simulink model "DPTThermalGaNModelSLX"  (R2018a)
settings: Solver=VariableStepAuto  StartTime=0.0  StopTime=8e-6  FixedStep=SampleTime  MinStep=0.5e-12  RelTol=1e-2  AbsTol=1e-9  EnableMultiTasking=on
values from neighbouring files (symbols this model uses):
  LoadCurrent = 15    [DPTThermalGaNModel.m]
  Rd = (3.6/4) * (0.95*0.82*(1 - (-0.0128*(Temp - 25))) * 18.2 / 295) + 1e-4    (= 0.11256119322)    [DPTThermalGaNModel.m]    (also in Thermal_CurrentVoltageGraph.m = (3.6/4) * (0.95*0.82*(1 - (-0.0128*(Temp(TempIndex) - 25))) )
  Rg = 1.5    [DPTThermalGaNModel.m]
  Roff = 2    [DPTThermalGaNModel.m]
  Ron = 10    [DPTThermalGaNModel.m]
  Rs = 3.6 * 0.238 * 0.82 * (1 - (-0.0128*(Temp - 25))) / 295 + 1e-4    (= 0.00629219525424)    [DPTThermalGaNModel.m]    (also in Thermal_CurrentVoltageGraph.m = 3.6 * 0.238 * 0.82 * (1 - (-0.0128*(Temp(TempIndex) - 25))) )
  Rss = 1e-3    (= 0.001)    [DPTThermalGaNModel.m]
  SampleTime = 5e-13    [DPTThermalGaNModel.m]
  Temp = 150    [DPTThermalGaNModel.m]    (also in Thermal_CurrentVoltageGraph.m = 25:25:150)
  Vdc = 400    [DPTThermalGaNModel.m]
  VpulseMax = 6    [DPTThermalGaNModel.m]
  VpulseMin = -3    [DPTThermalGaNModel.m]
undefined symbols (not defined in the file or in its folder): DiscIntNeverNeededParam, DT, T_ON
libraries: elec_lib x62, nesl_utility x33, fl_lib x27, simulink x2
(part 1 of 3)
settings Model: Creator=ugurm  LastModifiedBy=Furkan
settings SolverCC: ShapePreserveControl=EnableAll
settings OptimizationCC: EfficientMapNaN2IntZero=off  LifeSpan=inf
settings DebuggingCC: SFUnexpectedBacktrackingDiag=warning  SFNoUnconditionalDefaultTransitionDiag=warning  SFExecutionAtInitializationDiag=none
settings HardwareCC: TargetBitPerPointer=64  TargetBitPerSizeT=64  TargetBitPerPtrDiffT=64  TargetLongLongMode=on  TargetIntDivRoundTo=Zero  TargetEndianess=LittleEndian  TargetWordSize=64  TargetHWDeviceType=MATLAB Host  ProdEqTarget=off
settings CodeAppCC: MaxIdLength=128  StateflowObjectComments=on
settings GRTTargetCC: TargetLangStandard=C89/C90 (ANSI)  CombineOutputUpdateFcns=off  GRTInterface=on
settings ConfigComp: CovMetricSettings=dw  CovHtmlReporting=on  CovSaveCumulativeToWorkspaceVar=on  CovSaveSingleToWorkspaceVar=on  CovExternalEMLEnable=off
settings SimscapeCC: SimscapeNormalizeSystem=off

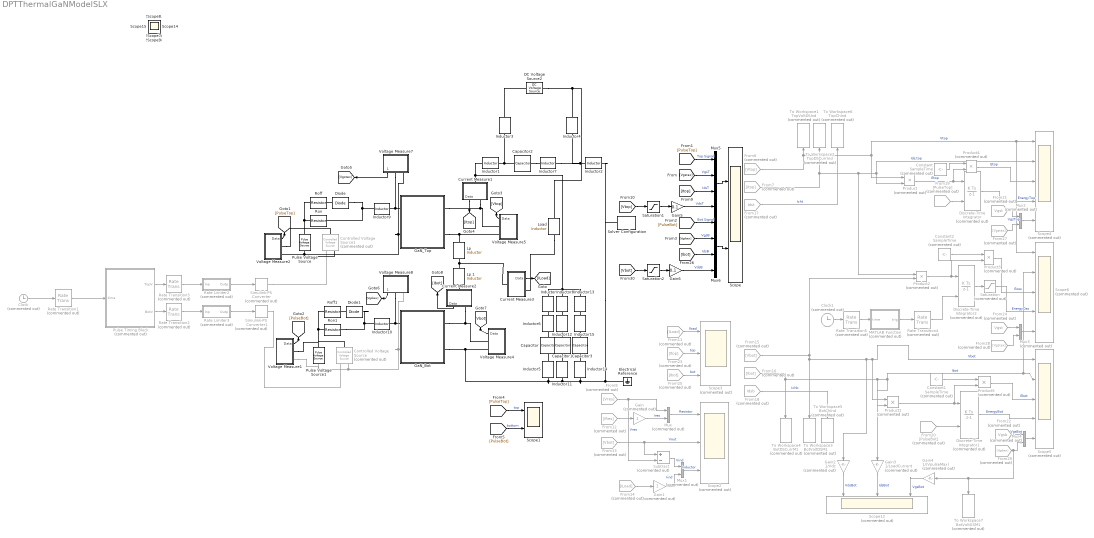
== system DPTThermalGaNModelSLX ==
  Capacitor : elec_lib/Passive Devices/Capacitor  enable_table=0  c=0.1e-6 F  Cvec=[1e-05, 1e-06] F  Vvec=[0, 10] V  CV_table_symmetry=1  C_tol=5  enable_C_tol=0  tol_distribution=1  nSigma=4  r=17.5e-3 Ohm  g=0 1/Ohm  enable_operating_limits=0  operating_limit_action=2  max_working_voltage_range=[-25, 25] V  power_rating=1 W  enable_faults=0  fault_action=1  Cscale_faulted=100  R_faulted=1e-3 Ohm  G_faulted=0 1/Ohm  tau_fault=1e-3 s  enable_temporal_fault=0  t_fault=1 s  enable_behavioral_fault=0  max_permissible_voltage_range=[-100, 100] V  t_fail_on_voltage=1 s  i_specify=off  i_priority=None  i=0 A  i_nominal_specify=off  i_nominal_unit=A  i_nominal_value=1  v_specify=off  v_priority=None  v=0 V  v_nominal_specify=off  v_nominal_unit=V  v_nominal_value=1  vc_specify=on  vc_priority=High  vc=Vdc V  vc_nominal_specify=off  vc_nominal_unit=V  vc_nominal_value=1
  Capacitor1 : elec_lib/Passive Devices/Capacitor  enable_table=0  c=0.1e-6 F  Cvec=[1e-05, 1e-06] F  Vvec=[0, 10] V  CV_table_symmetry=1  C_tol=5  enable_C_tol=0  tol_distribution=1  nSigma=4  r=17.5e-3 Ohm  g=0 1/Ohm  enable_operating_limits=0  operating_limit_action=2  max_working_voltage_range=[-25, 25] V  power_rating=1 W  enable_faults=0  fault_action=1  Cscale_faulted=100  R_faulted=1e-3 Ohm  G_faulted=0 1/Ohm  tau_fault=1e-3 s  enable_temporal_fault=0  t_fault=1 s  enable_behavioral_fault=0  max_permissible_voltage_range=[-100, 100] V  t_fail_on_voltage=1 s  i_specify=off  i_priority=None  i=0 A  i_nominal_specify=off  i_nominal_unit=A  i_nominal_value=1  v_specify=off  v_priority=None  v=0 V  v_nominal_specify=off  v_nominal_unit=V  v_nominal_value=1  vc_specify=on  vc_priority=High  vc=Vdc V  vc_nominal_specify=off  vc_nominal_unit=V  vc_nominal_value=1
  Capacitor2 : elec_lib/Passive Devices/Capacitor  enable_table=0  c=C F  Cvec=[ 1e-5 1e-6 ] F  Vvec=[ 0 10 ] V  CV_table_symmetry=1  C_tol=5  enable_C_tol=0  tol_distribution=1  nSigma=4  r=Resr Ohm  g=0 1/Ohm  enable_operating_limits=0  operating_limit_action=2  max_working_voltage_range=[ -25 25 ] V  power_rating=1 W  enable_faults=0  fault_action=1  Cscale_faulted=100  R_faulted=0.001 Ohm  G_faulted=0 1/Ohm  tau_fault=0.001 s  enable_temporal_fault=0  t_fault=1 s  enable_behavioral_fault=0  max_permissible_voltage_range=[ -100 100 ] V  t_fail_on_voltage=1 s  i_specify=off  i_priority=None  i=0 A  i_nominal_specify=off  i_nominal_unit=A  i_nominal_value=1  v_specify=off  v_priority=None  v=0 V  v_nominal_specify=off  v_nominal_unit=V  v_nominal_value=1  vc_specify=on  vc_priority=High  vc=Vdc V  vc_nominal_specify=off  vc_nominal_unit=V  vc_nominal_value=1
  Capacitor3 : elec_lib/Passive Devices/Capacitor  enable_table=0  c=0.1e-6 F  Cvec=[1e-05, 1e-06] F  Vvec=[0, 10] V  CV_table_symmetry=1  C_tol=5  enable_C_tol=0  tol_distribution=1  nSigma=4  r=17.5e-3 Ohm  g=0 1/Ohm  enable_operating_limits=0  operating_limit_action=2  max_working_voltage_range=[-25, 25] V  power_rating=1 W  enable_faults=0  fault_action=1  Cscale_faulted=100  R_faulted=1e-3 Ohm  G_faulted=0 1/Ohm  tau_fault=1e-3 s  enable_temporal_fault=0  t_fault=1 s  enable_behavioral_fault=0  max_permissible_voltage_range=[-100, 100] V  t_fail_on_voltage=1 s  i_specify=off  i_priority=None  i=0 A  i_nominal_specify=off  i_nominal_unit=A  i_nominal_value=1  v_specify=off  v_priority=None  v=0 V  v_nominal_specify=off  v_nominal_unit=V  v_nominal_value=1  vc_specify=on  vc_priority=High  vc=Vdc V  vc_nominal_specify=off  vc_nominal_unit=V  vc_nominal_value=1
  Clock : Clock  Commented=on
  Clock1 : Clock  Commented=on
  Constant : Constant  Commented=on  Value=SampleTime
  Constant1 : Constant  Commented=on  Value=SampleTime
  Constant2 : Constant  Commented=on  Value=SampleTime
  Controlled Voltage Source : fl_lib/Electrical/Electrical Sources/Controlled Voltage Source  Commented=on
  Controlled Voltage Source1 : fl_lib/Electrical/Electrical Sources/Controlled Voltage Source  Commented=on
  Current Measure1 : Subsystem
  Current Measure2 : Subsystem
  Current Measure3 : Subsystem
  DC Voltage Source2 : elec_lib/Additional Components/SPICE-Compatible Components/Sources/DC Voltage Source  DC=Vdc V
      settings: SourceProductName=Simscape Electronics  SourceProductBaseCode=SN
  Diode : elec_lib/Semiconductor Devices/Diode  ModelType=1  Vf=0.3 V  Ron=15e-3 Ohm  Goff=1e-8 S  Rz=0.3 Ohm  Vz=50 V  C_PWL=5 pF  prmExp=1  I12=[ 0.0137 0.545 ] A  V12=[ 0.6 0.7 ] V  I1=0.0137 A  V1=0.6 V  IS=1e-12 A  ec=1  RS=0.01 Ohm  Tmeas=25 degC  BV=Inf V  C_param=1  CJ0=5 pF  VJ=1 V  Mgrad=0.5  Vvec=[ 0.1 10 100 ] V  Cvec=[ 3.5 1 0.4 ] pF  FC=0.5  Q_param=1  Irrm=-7.15 A  iF=4 A  didt=-750 A/us  trr=115 ns  TT=50 ns  tau=100 ns  T_param=1  IS_T2=1.25e-7 A  I1_T2=0.245 A  V1_T2=0.5 V  Tmeas2=125 degC  EG_param=1  EG=1.11 eV  XTI_param=1  XTI=3  dBVdT=0 V/K  Tdevice=25 degC  i_capacitor_specify=off  i_capacitor_priority=High  i_capacitor=0 A  i_capacitor_nominal_specify=off  i_capacitor_nominal_unit=A  i_capacitor_nominal_value=1  v_capacitor_specify=off  v_capacitor_priority=None  v_capacitor=0 V  v_capacitor_nominal_specify=off  v_capacitor_nominal_unit=V  v_capacitor_nominal_value=1  Rth=[ 0 10 ] K/W  thermal_mass_parameterization=1  thermal_mass=[ 0 1 ] J/K  thermal_time_constant=[ 0 10 ] s  thermal_mass_initial_temperatures=[ 25 25 ] degC
      settings: SourceProductName=Simscape Electronics  SourceProductBaseCode=SN
  Diode1 : elec_lib/Semiconductor Devices/Diode  ModelType=1  Vf=0.3 V  Ron=15e-3 Ohm  Goff=1e-8 S  Rz=0.3 Ohm  Vz=50 V  C_PWL=5 pF  prmExp=1  I12=[ 0.0137 0.545 ] A  V12=[ 0.6 0.7 ] V  I1=0.0137 A  V1=0.6 V  IS=1e-12 A  ec=1  RS=0.01 Ohm  Tmeas=25 degC  BV=Inf V  C_param=1  CJ0=5 pF  VJ=1 V  Mgrad=0.5  Vvec=[ 0.1 10 100 ] V  Cvec=[ 3.5 1 0.4 ] pF  FC=0.5  Q_param=1  Irrm=-7.15 A  iF=4 A  didt=-750 A/us  trr=115 ns  TT=50 ns  tau=100 ns  T_param=1  IS_T2=1.25e-7 A  I1_T2=0.245 A  V1_T2=0.5 V  Tmeas2=125 degC  EG_param=1  EG=1.11 eV  XTI_param=1  XTI=3  dBVdT=0 V/K  Tdevice=25 degC  i_capacitor_specify=off  i_capacitor_priority=High  i_capacitor=0 A  i_capacitor_nominal_specify=off  i_capacitor_nominal_unit=A  i_capacitor_nominal_value=1  v_capacitor_specify=off  v_capacitor_priority=None  v_capacitor=0 V  v_capacitor_nominal_specify=off  v_capacitor_nominal_unit=V  v_capacitor_nominal_value=1  Rth=[ 0 10 ] K/W  thermal_mass_parameterization=1  thermal_mass=[ 0 1 ] J/K  thermal_time_constant=[ 0 10 ] s  thermal_mass_initial_temperatures=[ 25 25 ] degC
      settings: SourceProductName=Simscape Electronics  SourceProductBaseCode=SN
  Discrete-Time Integrator : DiscreteIntegrator  Commented=on  ExternalReset=either  SampleTime=-1  ICPrevOutput=DiscIntNeverNeededParam  ICPrevScaledInput=DiscIntNeverNeededParam
  Discrete-Time Integrator1 : DiscreteIntegrator  Commented=on  ExternalReset=either  SampleTime=-1  ICPrevOutput=DiscIntNeverNeededParam  ICPrevScaledInput=DiscIntNeverNeededParam
  Discrete-Time Integrator2 : DiscreteIntegrator  Commented=on  ExternalReset=either  SampleTime=-1  ICPrevOutput=DiscIntNeverNeededParam  ICPrevScaledInput=DiscIntNeverNeededParam
  Electrical Reference : fl_lib/Electrical/Electrical Elements/Electrical Reference
  From11 : From  Commented=on  GotoTag=ILoad
  From12 : From  Commented=on  GotoTag=IRes
  From13 : From  Commented=on  GotoTag=Vbot
  From14 : From  Commented=on  GotoTag=ILoad
  From15 : From  Commented=on  GotoTag=Vbot
  From16 : From  Commented=on  GotoTag=Ibot
  From17 : From  Commented=on  GotoTag=Idst  TagVisibility=global
  From18 : From  Commented=on  GotoTag=Idsb  TagVisibility=global
  From19 : From  Commented=on  GotoTag=PulseTop
  From20 : From  Commented=on  GotoTag=PulseBot
  From21 : From  Commented=on  GotoTag=Vgst  TagVisibility=global
  From22 : From  Commented=on  GotoTag=Vgsb  TagVisibility=global
  From23 : From  Commented=on  GotoTag=Itop
  From24 : From  Commented=on  GotoTag=Vgst  TagVisibility=global
  From25 : From  Commented=on  GotoTag=Ibot
  From27 : From  Commented=on  GotoTag=Vgstex
  From28 : From  Commented=on  GotoTag=Vgstex
  From29 : From  Commented=on  GotoTag=Vgsbex
  From6 : From  Commented=on  GotoTag=Vtop
  From7 : From  Commented=on  GotoTag=Itop
  From8 : From  Commented=on  GotoTag=Vres
  GaN_Bot : Subsystem
  GaN_Top : Subsystem
  Gain : Gain  Commented=on
  Gain1 : Gain  Commented=on
  Gain2 : Gain  Commented=on  Gain=1/Vdc
  Gain3 : Gain  Commented=on  Gain=1/LoadCurrent
  Gain4 : Gain  Commented=on  Gain=1/(VpulseMax)
  Gain5 : Gain  Gain=0.1
  Gain6 : Gain  Gain=0.1
  Inductor : elec_lib/Passive Devices/Inductor  l=10e-9 H  L_tol=20  enable_L_tol=0  tol_distribution=1  nSigma=4  r=0 Ohm  g=1e-9 1/Ohm  enable_operating_limits=0  operating_limit_action=2  max_working_current=1 A  power_rating=1 W  enable_faults=0  fault_action=1  lambdaPercent=50  k_faulted=0.9999  turnsShort=0  openCct=0  groundShort=0  groundShortG=0 1/Ohm  tau_fault=1e-3 s  enable_temporal_fault=0  t_fault=1 s  enable_behavioral_fault=0  max_permissible_voltage=100 V  n_fail_on_voltage=1  max_permissible_current=1 A  t_fail_on_current=1 s  i_L_specify=off  i_L_priority=High  i_L=0 A  i_L_nominal_specify=off  i_L_nominal_unit=A  i_L_nominal_value=1
      settings: SourceProductName=Simscape Electronics  SourceProductBaseCode=SN
  Inductor1 : elec_lib/Passive Devices/Inductor  l=7.14e-9 H  L_tol=20  enable_L_tol=0  tol_distribution=1  nSigma=4  r=0 Ohm  g=1e-9 1/Ohm  enable_operating_limits=0  operating_limit_action=2  max_working_current=1 A  power_rating=1 W  enable_faults=0  fault_action=1  lambdaPercent=50  k_faulted=0.9999  turnsShort=0  openCct=0  groundShort=0  groundShortG=0 1/Ohm  tau_fault=0.001 s  enable_temporal_fault=0  t_fault=1 s  enable_behavioral_fault=0  max_permissible_voltage=100 V  n_fail_on_voltage=1  max_permissible_current=1 A  t_fail_on_current=1 s  i_L_specify=off  i_L_priority=High  i_L=0 A  i_L_nominal_specify=off  i_L_nominal_unit=A  i_L_nominal_value=1
      settings: SourceProductName=Simscape Electronics  SourceProductBaseCode=SN
  Inductor10 : elec_lib/Passive Devices/Inductor  l=Lgex H  L_tol=20  enable_L_tol=0  tol_distribution=1  nSigma=4  r=0 Ohm  g=1e-9 1/Ohm  enable_operating_limits=0  operating_limit_action=1  max_working_current=1 A  power_rating=1 W  enable_faults=0  fault_action=1  lambdaPercent=50  k_faulted=0.9999  turnsShort=0  openCct=0  groundShort=0  groundShortG=0 1/Ohm  tau_fault=0.001 s  enable_temporal_fault=0  t_fault=1 s  enable_behavioral_fault=0  max_permissible_voltage=100 V  n_fail_on_voltage=1  max_permissible_current=1 A  t_fail_on_current=1 s  i_L_specify=on  i_L_priority=High  i_L=0 A  i_L_nominal_specify=off  i_L_nominal_unit=A  i_L_nominal_value=1
      settings: SourceProductName=Simscape Electronics  SourceProductBaseCode=SN
  Inductor11 : elec_lib/Passive Devices/Inductor  l=12e-9 H  L_tol=20  enable_L_tol=0  tol_distribution=1  nSigma=4  r=0 Ohm  g=1e-9 1/Ohm  enable_operating_limits=0  operating_limit_action=2  max_working_current=1 A  power_rating=1 W  enable_faults=0  fault_action=1  lambdaPercent=50  k_faulted=0.9999  turnsShort=0  openCct=0  groundShort=0  groundShortG=0 1/Ohm  tau_fault=1e-3 s  enable_temporal_fault=0  t_fault=1 s  enable_behavioral_fault=0  max_permissible_voltage=100 V  n_fail_on_voltage=1  max_permissible_current=1 A  t_fail_on_current=1 s  i_L_specify=off  i_L_priority=High  i_L=0 A  i_L_nominal_specify=off  i_L_nominal_unit=A  i_L_nominal_value=1
      settings: SourceProductName=Simscape Electronics  SourceProductBaseCode=SN
  Inductor12 : elec_lib/Passive Devices/Inductor  l=0.75e-9 H  L_tol=20  enable_L_tol=0  tol_distribution=1  nSigma=4  r=0 Ohm  g=1e-9 1/Ohm  enable_operating_limits=0  operating_limit_action=2  max_working_current=1 A  power_rating=1 W  enable_faults=0  fault_action=1  lambdaPercent=50  k_faulted=0.9999  turnsShort=0  openCct=0  groundShort=0  groundShortG=0 1/Ohm  tau_fault=1e-3 s  enable_temporal_fault=0  t_fault=1 s  enable_behavioral_fault=0  max_permissible_voltage=100 V  n_fail_on_voltage=1  max_permissible_current=1 A  t_fail_on_current=1 s  i_L_specify=off  i_L_priority=High  i_L=0 A  i_L_nominal_specify=off  i_L_nominal_unit=A  i_L_nominal_value=1
      settings: SourceProductName=Simscape Electronics  SourceProductBaseCode=SN
  Inductor13 : elec_lib/Passive Devices/Inductor  l=10e-9 H  L_tol=20  enable_L_tol=0  tol_distribution=1  nSigma=4  r=0 Ohm  g=1e-9 1/Ohm  enable_operating_limits=0  operating_limit_action=2  max_working_current=1 A  power_rating=1 W  enable_faults=0  fault_action=1  lambdaPercent=50  k_faulted=0.9999  turnsShort=0  openCct=0  groundShort=0  groundShortG=0 1/Ohm  tau_fault=1e-3 s  enable_temporal_fault=0  t_fault=1 s  enable_behavioral_fault=0  max_permissible_voltage=100 V  n_fail_on_voltage=1  max_permissible_current=1 A  t_fail_on_current=1 s  i_L_specify=off  i_L_priority=High  i_L=0 A  i_L_nominal_specify=off  i_L_nominal_unit=A  i_L_nominal_value=1
      settings: SourceProductName=Simscape Electronics  SourceProductBaseCode=SN
  Inductor14 : elec_lib/Passive Devices/Inductor  l=12e-9 H  L_tol=20  enable_L_tol=0  tol_distribution=1  nSigma=4  r=0 Ohm  g=1e-9 1/Ohm  enable_operating_limits=0  operating_limit_action=2  max_working_current=1 A  power_rating=1 W  enable_faults=0  fault_action=1  lambdaPercent=50  k_faulted=0.9999  turnsShort=0  openCct=0  groundShort=0  groundShortG=0 1/Ohm  tau_fault=1e-3 s  enable_temporal_fault=0  t_fault=1 s  enable_behavioral_fault=0  max_permissible_voltage=100 V  n_fail_on_voltage=1  max_permissible_current=1 A  t_fail_on_current=1 s  i_L_specify=off  i_L_priority=High  i_L=0 A  i_L_nominal_specify=off  i_L_nominal_unit=A  i_L_nominal_value=1
      settings: SourceProductName=Simscape Electronics  SourceProductBaseCode=SN
  Inductor15 : elec_lib/Passive Devices/Inductor  l=0.75e-9 H  L_tol=20  enable_L_tol=0  tol_distribution=1  nSigma=4  r=0 Ohm  g=1e-9 1/Ohm  enable_operating_limits=0  operating_limit_action=2  max_working_current=1 A  power_rating=1 W  enable_faults=0  fault_action=1  lambdaPercent=50  k_faulted=0.9999  turnsShort=0  openCct=0  groundShort=0  groundShortG=0 1/Ohm  tau_fault=1e-3 s  enable_temporal_fault=0  t_fault=1 s  enable_behavioral_fault=0  max_permissible_voltage=100 V  n_fail_on_voltage=1  max_permissible_current=1 A  t_fail_on_current=1 s  i_L_specify=off  i_L_priority=High  i_L=0 A  i_L_nominal_specify=off  i_L_nominal_unit=A  i_L_nominal_value=1
      settings: SourceProductName=Simscape Electronics  SourceProductBaseCode=SN
  Inductor2 : elec_lib/Passive Devices/Inductor  l=5.658e-9 H  L_tol=20  enable_L_tol=0  tol_distribution=1  nSigma=4  r=0.025 Ohm  g=1e-9 1/Ohm  enable_operating_limits=0  operating_limit_action=2  max_working_current=1 A  power_rating=1 W  enable_faults=0  fault_action=1  lambdaPercent=50  k_faulted=0.9999  turnsShort=0  openCct=0  groundShort=0  groundShortG=0 1/Ohm  tau_fault=0.001 s  enable_temporal_fault=0  t_fault=1 s  enable_behavioral_fault=0  max_permissible_voltage=100 V  n_fail_on_voltage=1  max_permissible_current=1 A  t_fail_on_current=1 s  i_L_specify=off  i_L_priority=None  i_L=0 A  i_L_nominal_specify=off  i_L_nominal_unit=A  i_L_nominal_value=1
      settings: SourceProductName=Simscape Electronics  SourceProductBaseCode=SN
  Inductor3 : elec_lib/Passive Devices/Inductor  l=29.8e-9 H  L_tol=20  enable_L_tol=0  tol_distribution=1  nSigma=4  r=0 Ohm  g=1e-9 1/Ohm  enable_operating_limits=0  operating_limit_action=2  max_working_current=1 A  power_rating=1 W  enable_faults=0  fault_action=1  lambdaPercent=50  k_faulted=0.9999  turnsShort=0  openCct=0  groundShort=0  groundShortG=0 1/Ohm  tau_fault=0.001 s  enable_temporal_fault=0  t_fault=1 s  enable_behavioral_fault=0  max_permissible_voltage=100 V  n_fail_on_voltage=1  max_permissible_current=1 A  t_fail_on_current=1 s  i_L_specify=on  i_L_priority=High  i_L=0 A  i_L_nominal_specify=off  i_L_nominal_unit=A  i_L_nominal_value=1
      settings: SourceProductName=Simscape Electronics  SourceProductBaseCode=SN
  Inductor4 : elec_lib/Passive Devices/Inductor  l=48.6e-9 H  L_tol=20  enable_L_tol=0  tol_distribution=1  nSigma=4  r=0 Ohm  g=1e-9 1/Ohm  enable_operating_limits=0  operating_limit_action=2  max_working_current=1 A  power_rating=1 W  enable_faults=0  fault_action=1  lambdaPercent=50  k_faulted=0.9999  turnsShort=0  openCct=0  groundShort=0  groundShortG=0 1/Ohm  tau_fault=0.001 s  enable_temporal_fault=0  t_fault=1 s  enable_behavioral_fault=0  max_permissible_voltage=100 V  n_fail_on_voltage=1  max_permissible_current=1 A  t_fail_on_current=1 s  i_L_specify=on  i_L_priority=High  i_L=0 A  i_L_nominal_specify=off  i_L_nominal_unit=A  i_L_nominal_value=1
      settings: SourceProductName=Simscape Electronics  SourceProductBaseCode=SN
  Inductor5 : elec_lib/Passive Devices/Inductor  l=12e-9 H  L_tol=20  enable_L_tol=0  tol_distribution=1  nSigma=4  r=0 Ohm  g=1e-9 1/Ohm  enable_operating_limits=0  operating_limit_action=2  max_working_current=1 A  power_rating=1 W  enable_faults=0  fault_action=1  lambdaPercent=50  k_faulted=0.9999  turnsShort=0  openCct=0  groundShort=0  groundShortG=0 1/Ohm  tau_fault=1e-3 s  enable_temporal_fault=0  t_fault=1 s  enable_behavioral_fault=0  max_permissible_voltage=100 V  n_fail_on_voltage=1  max_permissible_current=1 A  t_fail_on_current=1 s  i_L_specify=off  i_L_priority=High  i_L=0 A  i_L_nominal_specify=off  i_L_nominal_unit=A  i_L_nominal_value=1
      settings: SourceProductName=Simscape Electronics  SourceProductBaseCode=SN
  Inductor6 : elec_lib/Passive Devices/Inductor  l=0.75e-9 H  L_tol=20  enable_L_tol=0  tol_distribution=1  nSigma=4  r=0 Ohm  g=1e-9 1/Ohm  enable_operating_limits=0  operating_limit_action=2  max_working_current=1 A  power_rating=1 W  enable_faults=0  fault_action=1  lambdaPercent=50  k_faulted=0.9999  turnsShort=0  openCct=0  groundShort=0  groundShortG=0 1/Ohm  tau_fault=1e-3 s  enable_temporal_fault=0  t_fault=1 s  enable_behavioral_fault=0  max_permissible_voltage=100 V  n_fail_on_voltage=1  max_permissible_current=1 A  t_fail_on_current=1 s  i_L_specify=off  i_L_priority=High  i_L=0 A  i_L_nominal_specify=off  i_L_nominal_unit=A  i_L_nominal_value=1
      settings: SourceProductName=Simscape Electronics  SourceProductBaseCode=SN
  Inductor7 : elec_lib/Passive Devices/Inductor  l=19e-9 H  L_tol=20  enable_L_tol=0  tol_distribution=1  nSigma=4  r=0 Ohm  g=1e-9 1/Ohm  enable_operating_limits=0  operating_limit_action=2  max_working_current=1 A  power_rating=1 W  enable_faults=0  fault_action=1  lambdaPercent=50  k_faulted=0.9999  turnsShort=0  openCct=0  groundShort=0  groundShortG=0 1/Ohm  tau_fault=0.001 s  enable_temporal_fault=0  t_fault=1 s  enable_behavioral_fault=0  max_permissible_voltage=100 V  n_fail_on_voltage=1  max_permissible_current=1 A  t_fail_on_current=1 s  i_L_specify=on  i_L_priority=High  i_L=0 A  i_L_nominal_specify=off  i_L_nominal_unit=A  i_L_nominal_value=1
      settings: SourceProductName=Simscape Electronics  SourceProductBaseCode=SN
  Inductor8 : elec_lib/Passive Devices/Inductor  l=10e-9 H  L_tol=20  enable_L_tol=0  tol_distribution=1  nSigma=4  r=0 Ohm  g=1e-9 1/Ohm  enable_operating_limits=0  operating_limit_action=2  max_working_current=1 A  power_rating=1 W  enable_faults=0  fault_action=1  lambdaPercent=50  k_faulted=0.9999  turnsShort=0  openCct=0  groundShort=0  groundShortG=0 1/Ohm  tau_fault=1e-3 s  enable_temporal_fault=0  t_fault=1 s  enable_behavioral_fault=0  max_permissible_voltage=100 V  n_fail_on_voltage=1  max_permissible_current=1 A  t_fail_on_current=1 s  i_L_specify=off  i_L_priority=High  i_L=0 A  i_L_nominal_specify=off  i_L_nominal_unit=A  i_L_nominal_value=1
      settings: SourceProductName=Simscape Electronics  SourceProductBaseCode=SN
  Inductor9 : elec_lib/Passive Devices/Inductor  l=Lgex H  L_tol=20  enable_L_tol=0  tol_distribution=1  nSigma=4  r=0 Ohm  g=1e-9 1/Ohm  enable_operating_limits=0  operating_limit_action=1  max_working_current=1 A  power_rating=1 W  enable_faults=0  fault_action=1  lambdaPercent=50  k_faulted=0.9999  turnsShort=0  openCct=0  groundShort=0  groundShortG=0 1/Ohm  tau_fault=0.001 s  enable_temporal_fault=0  t_fault=1 s  enable_behavioral_fault=0  max_permissible_voltage=100 V  n_fail_on_voltage=1  max_permissible_current=1 A  t_fail_on_current=1 s  i_L_specify=on  i_L_priority=High  i_L=0 A  i_L_nominal_specify=off  i_L_nominal_unit=A  i_L_nominal_value=1
      settings: SourceProductName=Simscape Electronics  SourceProductBaseCode=SN
  Load : elec_lib/Passive Devices/Inductor  l=Lload H  L_tol=20  enable_L_tol=0  tol_distribution=1  nSigma=4  r=0 Ohm  g=1e-9 1/Ohm  enable_operating_limits=0  operating_limit_action=2  max_working_current=1 A  power_rating=1 W  enable_faults=0  fault_action=1  lambdaPercent=50  k_faulted=0.9999  turnsShort=0  openCct=0  groundShort=0  groundShortG=0 1/Ohm  tau_fault=0.001 s  enable_temporal_fault=0  t_fault=1 s  enable_behavioral_fault=0  max_permissible_voltage=100 V  n_fail_on_voltage=1  max_permissible_current=1 A  t_fail_on_current=1 s  i_L_specify=on  i_L_priority=High  i_L=InitialCurrent A  i_L_nominal_specify=off  i_L_nominal_unit=A  i_L_nominal_value=1
      settings: SourceProductName=Simscape Electronics  SourceProductBaseCode=SN
  "Lp " : elec_lib/Passive Devices/Inductor  l=3.724e-9 H  L_tol=20  enable_L_tol=0  tol_distribution=1  nSigma=4  r=0 Ohm  g=1e-9 1/Ohm  enable_operating_limits=0  operating_limit_action=2  max_working_current=1 A  power_rating=1 W  enable_faults=0  fault_action=1  lambdaPercent=50  k_faulted=0.9999  turnsShort=0  openCct=0  groundShort=0  groundShortG=0 1/Ohm  tau_fault=0.001 s  enable_temporal_fault=0  t_fault=1 s  enable_behavioral_fault=0  max_permissible_voltage=100 V  n_fail_on_voltage=1  max_permissible_current=1 A  t_fail_on_current=1 s  i_L_specify=off  i_L_priority=High  i_L=CurrDSTop A  i_L_nominal_specify=off  i_L_nominal_unit=A  i_L_nominal_value=1
      settings: SourceProductName=Simscape Electronics  SourceProductBaseCode=SN
  Lp 1 : elec_lib/Passive Devices/Inductor  l=3.724e-9 H  L_tol=20  enable_L_tol=0  tol_distribution=1  nSigma=4  r=0 Ohm  g=1e-9 1/Ohm  enable_operating_limits=0  operating_limit_action=2  max_working_current=1 A  power_rating=1 W  enable_faults=0  fault_action=1  lambdaPercent=50  k_faulted=0.9999  turnsShort=0  openCct=0  groundShort=0  groundShortG=0 1/Ohm  tau_fault=0.001 s  enable_temporal_fault=0  t_fault=1 s  enable_behavioral_fault=0  max_permissible_voltage=100 V  n_fail_on_voltage=1  max_permissible_current=1 A  t_fail_on_current=1 s  i_L_specify=off  i_L_priority=High  i_L=CurrDSTop A  i_L_nominal_specify=off  i_L_nominal_unit=A  i_L_nominal_value=1
      settings: SourceProductName=Simscape Electronics  SourceProductBaseCode=SN
  MATLAB Function : MATLAB Function  Commented=on  TreatAsAtomicUnit=on  SystemSampleTime=1e-10
  Mux{,1..4} (5 alike) : Mux  Commented=on  Inputs=2
  Mux5 : Mux
  Mux6 : Mux
  Product{,1..5} (6 alike) : Product  Commented=on
  Pulse Timing Block : MATLAB Function  Commented=on  TreatAsAtomicUnit=on  SystemSampleTime=1e-9
  Pulse Voltage Source : elec_lib/Additional Components/SPICE-Compatible Components/Sources/Pulse Voltage Source  V1=VpulseMin V  V2=VpulseMax V  TD=DT s  TR=RiseTime s  TF=FallTime s  PW=T_ON-2*DT s  PER=T_P s
      settings: SourceProductName=Simscape Electronics  SourceProductBaseCode=SN
  Pulse Voltage Source1 : elec_lib/Additional Components/SPICE-Compatible Components/Sources/Pulse Voltage Source  V1=VpulseMax V  V2=VpulseMin V  TD=0 s  TR=RiseTime s  TF=FallTime s  PW=T_ON s  PER=T_P s
      settings: SourceProductName=Simscape Electronics  SourceProductBaseCode=SN
  Rate Limiter2 : Subsystem  Commented=on
  Rate Limiter3 : Subsystem  Commented=on
  Rate Transition1 : RateTransition  Commented=on  OutPortSampleTime=1e-9
  Rate Transition2 : RateTransition  Commented=on  OutPortSampleTime=SampleTime
  Rate Transition3 : RateTransition  Commented=on  OutPortSampleTime=SampleTime
  Rate Transition4 : RateTransition  Commented=on  OutPortSampleTime=SampleTime
  Rate Transition5 : RateTransition  Commented=on  OutPortSampleTime=1e-10
  Roff : elec_lib/Passive Devices/Resistor  R=Roff Ohm  R_tol=5  enable_R_tol=0  tol_distribution=1  nSigma=4  enable_operating_limits=0  operating_limit_action=2  max_working_voltage=100 V  power_rating=1 W  enable_faults=0  fault_action=1  R_faulted=Inf Ohm  enable_temporal_fault=0  t_fault=1 s  enable_behavioral_fault=0  max_permissible_current=1 A  t_fail_on_current=1 s  noise_mode=0  sample_time=0.001 s  repeatability=1  auto_seed=2348838240  user_seed=0  Tdevice=25 degC  alpha=3.93e-3 1/K  Tmeas=25 degC  thermal_mass=100 J/K  power_derating_T1=70 degC  power_derating_T2=155 degC  operating_temperature_range_vec=[-50, 150] degC  temperature_specify=off  temperature_priority=High  temperature=298.15 K  temperature_nominal_specify=off  temperature_nominal_unit=K  temperature_nominal_value=1
  Roff1 : elec_lib/Passive Devices/Resistor  R=Roff Ohm  R_tol=5  enable_R_tol=0  tol_distribution=1  nSigma=4  enable_operating_limits=0  operating_limit_action=2  max_working_voltage=100 V  power_rating=1 W  enable_faults=0  fault_action=1  R_faulted=Inf Ohm  enable_temporal_fault=0  t_fault=1 s  enable_behavioral_fault=0  max_permissible_current=1 A  t_fail_on_current=1 s  noise_mode=0  sample_time=0.001 s  repeatability=1  auto_seed=4112460543  user_seed=0  Tdevice=25 degC  alpha=3.93e-3 1/K  Tmeas=25 degC  thermal_mass=100 J/K  power_derating_T1=70 degC  power_derating_T2=155 degC  operating_temperature_range_vec=[-50, 150] degC  temperature_specify=off  temperature_priority=High  temperature=298.15 K  temperature_nominal_specify=off  temperature_nominal_unit=K  temperature_nominal_value=1
  Ron : elec_lib/Passive Devices/Resistor  R=Ron Ohm  R_tol=5  enable_R_tol=0  tol_distribution=1  nSigma=4  enable_operating_limits=0  operating_limit_action=2  max_working_voltage=100 V  power_rating=1 W  enable_faults=0  fault_action=1  R_faulted=Inf Ohm  enable_temporal_fault=0  t_fault=1 s  enable_behavioral_fault=0  max_permissible_current=1 A  t_fail_on_current=1 s  noise_mode=0  sample_time=0.001 s  repeatability=1  auto_seed=4144164703  user_seed=0  Tdevice=25 degC  alpha=3.93e-3 1/K  Tmeas=25 degC  thermal_mass=100 J/K  power_derating_T1=70 degC  power_derating_T2=155 degC  operating_temperature_range_vec=[-50, 150] degC  temperature_specify=off  temperature_priority=High  temperature=298.15 K  temperature_nominal_specify=off  temperature_nominal_unit=K  temperature_nominal_value=1
  Ron1 : elec_lib/Passive Devices/Resistor  R=Ron Ohm  R_tol=5  enable_R_tol=0  tol_distribution=1  nSigma=4  enable_operating_limits=0  operating_limit_action=2  max_working_voltage=100 V  power_rating=1 W  enable_faults=0  fault_action=1  R_faulted=Inf Ohm  enable_temporal_fault=0  t_fault=1 s  enable_behavioral_fault=0  max_permissible_current=1 A  t_fail_on_current=1 s  noise_mode=0  sample_time=0.001 s  repeatability=1  auto_seed=676943032  user_seed=0  Tdevice=25 degC  alpha=3.93e-3 1/K  Tmeas=25 degC  thermal_mass=100 J/K  power_derating_T1=70 degC  power_derating_T2=155 degC  operating_temperature_range_vec=[-50, 150] degC  temperature_specify=off  temperature_priority=High  temperature=298.15 K  temperature_nominal_specify=off  temperature_nominal_unit=K  temperature_nominal_value=1
  Saturation : Saturate  Commented=on  UpperLimit=100e-6  LowerLimit=0
  Saturation1 : Saturate  UpperLimit=1.5*Vdc  LowerLimit=-1.5*Vdc
  Saturation2 : Saturate  UpperLimit=1.5*Vdc  LowerLimit=-1.5*Vdc
  Scope : Scope  NumInputPorts=2
  Scope1 : Scope  NumInputPorts=2
  Scope12 : Scope  Commented=on  NumInputPorts=3
  Scope2 : Scope  Commented=on  NumInputPorts=3
  Scope3 : Scope  Commented=on  NumInputPorts=3
  Scope4 : Scope  Commented=on  NumInputPorts=5
  Scope5 : Scope  Commented=on  NumInputPorts=5
  Scope6 : Scope  Commented=on  NumInputPorts=5
  Simulink-PS Converter : nesl_utility/Simulink-PS Converter  Commented=on  PhysicalDomain=network_engine_domain  SubClassName=ps_input  LeftPortType=input  RightPortType=output  PseudoPeriodic=off  Frequencies=[]  NoiseDistribution=none  NoiseParameters=[]  Unit=1  AffineConversion=off  FilteringAndDerivatives=zero  SimscapeFilterOrder=1  InputFilterTimeConstant=0.001  UdotUserProvided=1
  Simulink-PS Converter1 : nesl_utility/Simulink-PS Converter  Commented=on  PhysicalDomain=network_engine_domain  SubClassName=ps_input  LeftPortType=input  RightPortType=output  PseudoPeriodic=off  Frequencies=[]  NoiseDistribution=none  NoiseParameters=[]  Unit=1  AffineConversion=off  FilteringAndDerivatives=zero  SimscapeFilterOrder=1  InputFilterTimeConstant=0.001  UdotUserProvided=1
  Solver Configuration : nesl_utility/Solver Configuration  PhysicalDomain=network_engine_domain  SubClassName=solver  LeftPortType=input  RightPortType=generic  Tones=[]  Harmonics=[]  SimulateNoise=off  Profile=off  UseLocalSampling=off  EnableSwitchedLinearOptims=on  FrequencyDomain=off  UseCCode=off  RelTol=0.001  AbsTol=1e-06  MinStep=1e-09  ToWorkspace=off  RevertToSquareIcSolve=off  NumHomotopyIterations=100  PhasorMode=off  PhasorModeNumHarmonics=1  DoDC=off  ResidualTolerance=1e-09  UseLocalSolver=on  LocalSolverChoice=NE_BACKWARD_EULER_ADVANCER  LocalSolverSampleTime=SampleTime  DoFixedCost=on  MaxNonlinIter=3  MaxModeIter=2  LinearAlgebra=Sparse  EquationFormulation=NE_TIME_EF  DelaysMemoryBudget=1024  AutomaticFiltering=on  FilteringTimeConstant=0.001
  Subtract : Sum  Commented=on  Inputs=+-
  To Workspace1 : ToWorkspace  Commented=on  VariableName=TopVoltDSInd  SampleTime=-1
      settings: Save2DSignal=2-D array (concatenate along first dimension)
  To Workspace2 : ToWorkspace  Commented=on  VariableName=TopDSCurrInd  SampleTime=-1
      settings: Save2DSignal=2-D array (concatenate along first dimension)
  To Workspace3 : ToWorkspace  Commented=on  VariableName=BotVoltDSM1  SampleTime=-1
      settings: Save2DSignal=2-D array (concatenate along first dimension)
  To Workspace4 : ToWorkspace  Commented=on  VariableName=BotDSCurrM1  SampleTime=-1
      settings: Save2DSignal=2-D array (concatenate along first dimension)
  To Workspace5 : ToWorkspace  Commented=on  VariableName=BotChInd  SampleTime=-1
      settings: Save2DSignal=2-D array (concatenate along first dimension)
  To Workspace6 : ToWorkspace  Commented=on  VariableName=TopChInd  SampleTime=-1
      settings: Save2DSignal=2-D array (concatenate along first dimension)
  To Workspace7 : ToWorkspace  Commented=on  VariableName=BotVoltGSM1  SampleTime=-1
      settings: Save2DSignal=2-D array (concatenate along first dimension)
  Voltage Measure1 : Subsystem
  Voltage Measure2 : Subsystem
  Voltage Measure4 : Subsystem
  Voltage Measure5 : Subsystem
  Voltage Measure7 : Subsystem
  Voltage Measure8 : Subsystem
  Scope{7..11,13..15} (8 alike) : Scope
  wires:
  Current Measure3/1(Data) -> [ILoad]
  From11/1 -> Scope3/1  "Iload"
  [PulseTop] -> Scope1/1  "top"
  [PulseBot] -> Scope1/2  "bottom"
  Voltage Measure2/1(Data) -> [PulseTop]
  Voltage Measure1/1(Data) -> [PulseBot]
  Voltage Measure4/1(Data) -> [Vbot]
  From8/1 -> Mux/1, Subtract/2  "Vres"
  From12/1 -> Gain/1
  Mux/1 -> Scope2/1  "Resistor"
  From13/1 -> Scope2/2, Subtract/1  "Vout"
  Mux1/1 -> Scope2/3  "Inductor"
  From14/1 -> Gain1/1
  Subtract/1 -> Mux1/1  "Vind"
  Gain/1 -> Mux/2  "Ires"
  Gain1/1 -> Mux1/2  "Iind"
  Voltage Measure5/1(Data) -> [Vtop]
  Current Measure1/1(Data) -> [Itop]
  Current Measure2/1(Data) -> [Ibot]
  From7/1 -> Product2/1, Scope4/2, Product/2, To Workspace2/1  "Ids,top"
  From18/1 -> To Workspace5/1  "Ichb"
  From16/1 -> To Workspace4/1, Gain3/1, Scope6/2, Scope5/2, Product1/2  "Ibot"
  From17/1 -> To Workspace6/1  "Icht"
  Clock/1 -> Rate Transition1/1
  Rate Transition1/1 -> Pulse Timing Block/1(time)
  Rate Transition2/1 -> Rate Limiter3/1(Inp)
  Rate Transition3/1 -> Rate Limiter2/1(Inp)
  Product/1 -> Product4/2, Discrete-Time Integrator/1  "Etop"
  From19/1 -> Discrete-Time Integrator/2
  Product1/1 -> Product5/2, Discrete-Time Integrator1/1
  From20/1 -> Discrete-Time Integrator1/2
  From6/1 -> To Workspace1/1, Scope6/1, Scope4/1, Product/1  "Vtop"
  From15/1 -> Product2/2, To Workspace3/1, Gain2/1, Scope5/1, Product1/1  "Vbot"
  Pulse Timing Block/1(TopV) -> Rate Transition3/1
  Pulse Timing Block/2(BotV) -> Rate Transition2/1
  Rate Limiter2/1(Outp) -> Simulink-PS Converter/1
  Rate Limiter3/1(Outp) -> Simulink-PS Converter1/1
  Product2/1 -> Product3/2, Discrete-Time Integrator2/1
  Discrete-Time Integrator2/1 -> Saturation/1
  Discrete-Time Integrator/1 -> Scope4/4  "EnergyTop"
  Discrete-Time Integrator1/1 -> Scope5/4  "EnergyBot"
  Saturation/1 -> Scope6/4  "EnergyOss"
  Clock1/1 -> Rate Transition5/1
  MATLAB Function/1(trig) -> Rate Transition4/1
  Rate Transition4/1 -> Discrete-Time Integrator2/2
  Rate Transition5/1 -> MATLAB Function/1(time)
  Product3/1 -> Scope6/3  "Eoss"
  Constant2/1 -> Product3/1
  Product4/1 -> Scope4/3  "Etop"
  Constant/1 -> Product4/1
  Product5/1 -> Scope5/3  "Ebot"
  Constant1/1 -> Product5/1
  From23/1 -> Scope3/2  "top"
  From25/1 -> Scope3/3  "bot"
  Gain2/1 -> Scope12/1  "VdsBot"
  Voltage Measure7/1(Data) -> [Vgstex]
  Voltage Measure8/1(Data) -> [Vgsbex]
  Mux2/1 -> Scope4/5
  From21/1 -> Mux2/1  "VgsTop"
  From27/1 -> Mux2/2
  Mux3/1 -> Scope6/5
  From24/1 -> Mux3/1
  From28/1 -> Mux3/2
  Mux4/1 -> Scope5/5
  From22/1 -> Mux4/1  "VgsBot"
  From29/1 -> Gain4/1, To Workspace7/1, Mux4/2
  Gain3/1 -> Scope12/2  "IdsBot"
  Gain4/1 -> Scope12/3  "VgsBot"
  [PulseBot] -> Mux6/1  "Bot Signal"
  [Vgsbex] -> Mux6/2  "VgsB"
  [Itop] -> Mux5/3  "IdsT"
  [Vtop] -> Saturation1/1
  [Ibot] -> Mux6/3  "IdsB"
  [Vbot] -> Saturation2/1
  [PulseTop] -> Mux5/1  "Top Signal"
  [Vgstex] -> Mux5/2  "VgsT"
  Mux5/1 -> Scope/1
  Mux6/1 -> Scope/2
  Gain5/1 -> Mux5/4  "VdsT"
  Gain6/1 -> Mux6/4  "VdsB"
  Saturation2/1 -> Gain6/1
  Saturation1/1 -> Gain5/1
  connections:
  Ron/RConn1 -- Controlled Voltage Source1/LConn1 -- Voltage Measure2/RConn1 -- Pulse Voltage Source/LConn1 -- Roff/RConn1
  Ron1/RConn1 -- Controlled Voltage Source/LConn1 -- Pulse Voltage Source1/LConn1 -- Voltage Measure1/RConn1 -- Roff1/RConn1
  Roff/LConn1 -- Diode/RConn1
  Roff1/LConn1 -- Diode1/RConn1
  GaN_Top/RConn1 -- Current Measure1/RConn1 -- Voltage Measure5/RConn1
  GaN_Bot/RConn1 -- Current Measure2/RConn1 -- Voltage Measure4/RConn1
  Simulink-PS Converter/RConn1 -- Controlled Voltage Source1/RConn1
  Simulink-PS Converter1/RConn1 -- Controlled Voltage Source/RConn1
  Diode1/LConn1 -- Ron1/LConn1 -- Inductor10/LConn1
  Inductor1/RConn1 -- Inductor3/LConn1 -- Capacitor2/LConn1
  Inductor2/LConn1 -- Inductor4/LConn1 -- Inductor7/RConn1
  Inductor3/RConn1 -- DC Voltage Source2/LConn1
  DC Voltage Source2/RConn1 -- Load/LConn1 -- Inductor4/RConn1
  Diode/LConn1 -- Inductor9/LConn1 -- Ron/LConn1
  Inductor9/RConn1 -- GaN_Top/LConn1 -- Voltage Measure7/RConn1
  Inductor10/RConn1 -- Voltage Measure8/RConn1 -- GaN_Bot/LConn1
  Current Measure3/LConn1 -- "Lp "/RConn1 -- Lp 1/LConn1
  Controlled Voltage Source/RConn2 -- Voltage Measure1/RConn2 -- Pulse Voltage Source1/RConn1 -- Voltage Measure8/RConn2 -- GaN_Bot/LConn2
  Load/RConn1 -- Current Measure3/RConn1
  Inductor2/RConn1 -- Solver Configuration/RConn1 -- Inductor14/RConn1 -- Inductor11/RConn1 -- Inductor5/RConn1 -- GaN_Bot/RConn2 -- Voltage Measure4/RConn2 -- Electrical Reference/LConn1
  Pulse Voltage Source/RConn1 -- Controlled Voltage Source1/RConn2 -- Voltage Measure2/RConn2 -- GaN_Top/LConn2 -- Voltage Measure7/RConn2
  Voltage Measure5/RConn2 -- "Lp "/LConn1 -- GaN_Top/RConn2
  Capacitor2/RConn1 -- Inductor7/LConn1
  Current Measure2/LConn1 -- Lp 1/RConn1
  Inductor5/LConn1 -- Capacitor/RConn1
  Inductor6/LConn1 -- Inductor/RConn1
  Inductor6/RConn1 -- Capacitor/LConn1
  Inductor11/LConn1 -- Capacitor1/RConn1
  Inductor12/LConn1 -- Inductor8/RConn1
  Inductor12/RConn1 -- Capacitor1/LConn1
  Inductor14/LConn1 -- Capacitor3/RConn1
  Inductor15/LConn1 -- Inductor13/RConn1
  Inductor15/RConn1 -- Capacitor3/LConn1
  Inductor1/LConn1 -- Inductor8/LConn1 -- Inductor13/LConn1 -- Inductor/LConn1 -- Current Measure1/LConn1

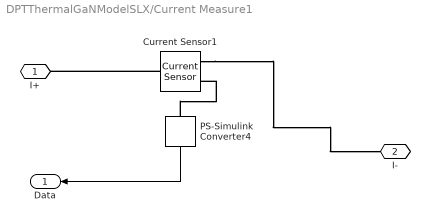
== system DPTThermalGaNModelSLX/Current Measure1 ==
  Current Sensor1 : fl_lib/Electrical/Electrical Sensors/Current Sensor
  PS-Simulink Converter4 : nesl_utility/PS-Simulink Converter  PhysicalDomain=network_engine_domain  SubClassName=ps_output  LeftPortType=input  RightPortType=output  PseudoPeriodic=off  Frequencies=[]  Unit=1  AffineConversion=off
  I+ : PMIOPort  Side=Left
  I- : PMIOPort  Port=2  Side=Right
  Data : Outport
  wires:
  PS-Simulink Converter4/1 -> Data/1
  connections:
  Current Sensor1/RConn2 -- I-/RConn1
  PS-Simulink Converter4/LConn1 -- Current Sensor1/RConn1
  Current Sensor1/LConn1 -- I+/RConn1

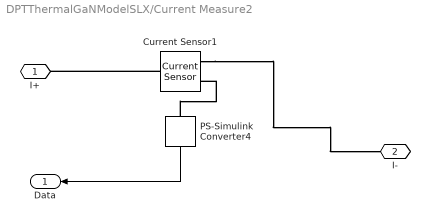
== system DPTThermalGaNModelSLX/Current Measure2 ==
  Current Sensor1 : fl_lib/Electrical/Electrical Sensors/Current Sensor
  PS-Simulink Converter4 : nesl_utility/PS-Simulink Converter  PhysicalDomain=network_engine_domain  SubClassName=ps_output  LeftPortType=input  RightPortType=output  PseudoPeriodic=off  Frequencies=[]  Unit=1  AffineConversion=off
  I+ : PMIOPort  Side=Left
  I- : PMIOPort  Port=2  Side=Right
  Data : Outport
  wires:
  PS-Simulink Converter4/1 -> Data/1
  connections:
  Current Sensor1/RConn2 -- I-/RConn1
  PS-Simulink Converter4/LConn1 -- Current Sensor1/RConn1
  Current Sensor1/LConn1 -- I+/RConn1

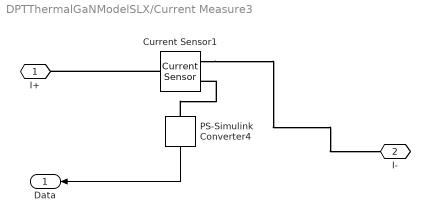
== system DPTThermalGaNModelSLX/Current Measure3 ==
  Current Sensor1 : fl_lib/Electrical/Electrical Sensors/Current Sensor
  PS-Simulink Converter4 : nesl_utility/PS-Simulink Converter  PhysicalDomain=network_engine_domain  SubClassName=ps_output  LeftPortType=input  RightPortType=output  PseudoPeriodic=off  Frequencies=[]  Unit=1  AffineConversion=off
  I+ : PMIOPort  Side=Left
  I- : PMIOPort  Port=2  Side=Right
  Data : Outport
  wires:
  PS-Simulink Converter4/1 -> Data/1
  connections:
  Current Sensor1/LConn1 -- I+/RConn1
  PS-Simulink Converter4/LConn1 -- Current Sensor1/RConn1
  Current Sensor1/RConn2 -- I-/RConn1
